simulink model "COMPONENT_model_SEME"  (R2019a)
settings: Solver=ode45  StartTime=0.0  StopTime=60  FixedStep=0.001  RelTol=1e-6  EnableMultiTasking=on
undefined symbols (not defined in the file or in its folder): d, Io, m, pm_0
settings Model: Creator=bhorton  LastModifiedBy=bhorton
settings SolverCC: ZeroCrossAlgorithm=Adaptive
settings DataIOCC: SaveOutput=off  SignalLogging=off  DSMLogging=off  VisualizeSimOutput=off  SaveTime=off  ReturnWorkspaceOutputs=off
settings OptimizationCC: LifeSpan=inf
settings DebuggingCC: AllowSymbolicDim=off  SFUnexpectedBacktrackingDiag=warning  SFNoUnconditionalDefaultTransitionDiag=warning  SFExecutionAtInitializationDiag=none  ArithmeticOperatorsInVariantConditions=warning
settings ModelReferenceCC: PropagateSignalLabelsOutOfModel=off
settings SFSimCC: SimUseLocalCustomCode=off
settings RTWCC: RTWUseLocalCustomCode=off
settings CodeAppCC: StateflowObjectComments=on
settings GRTTargetCC: TargetLangStandard=C89/C90 (ANSI)
settings ConfigComp: CovMetricSettings=dw  CovHtmlReporting=on  CovSaveCumulativeToWorkspaceVar=on  CovSaveSingleToWorkspaceVar=on  CovExternalEMLEnable=off
settings SimscapeCC: SimscapeNormalizeSystem=off

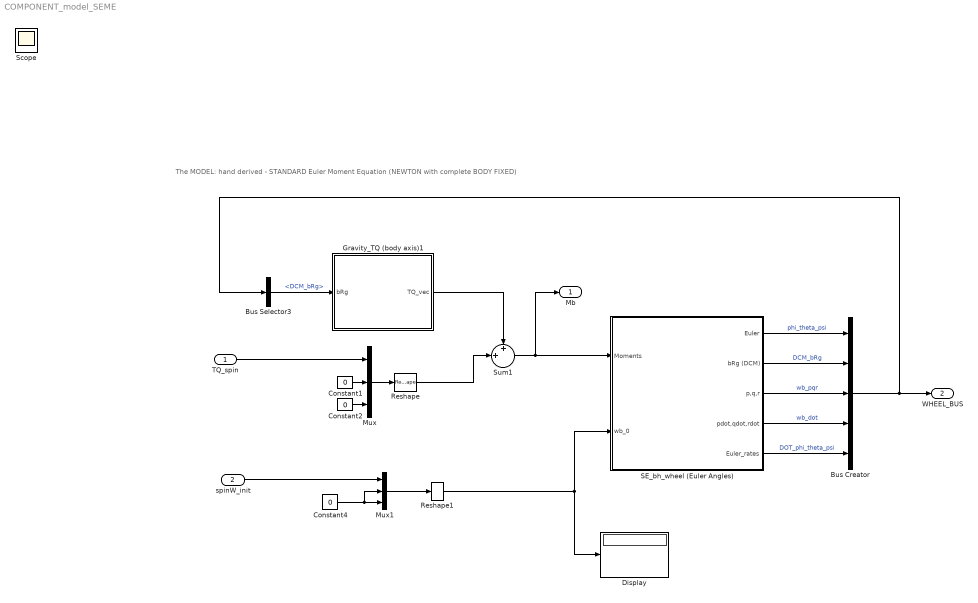
== system COMPONENT_model_SEME ==
  note: The MODEL: hand derived - STANDARD Euler Moment Equation (NEWTON with complete BODY FIXED)
  TQ_spin : Inport
  spinW_init : Inport  Port=2
  Bus Creator : BusCreator  Inputs=5
  Bus Selector3 : BusSelector  OutputSignals=DCM_bRg
  Constant1 : Constant  Value=0
  Constant2 : Constant  Value=0
  Constant4 : Constant  Value=0
  Display : Display
  Gravity_TQ (body axis)1 : Subsystem
  Mux : Mux  Inputs=3
  Mux1 : Mux  Inputs=3
  Reshape : Reshape  OutputDimensionality=Column vector (2-D)
  Reshape1 : Reshape  OutputDimensionality=Column vector (2-D)
  SE_bh_wheel (Euler Angles) : Subsystem  mask(bh_wheel_EoM (Body Axis)){inertia_0=Io, wb_0=[0;0;0], eul_0=deg2rad([0;0;0])}
      mask prompts: inertia_0 "Vehicle Inertia about TOWER pivot point, [kg.m^2]"; wb_0 "Initial body FRAME rotation rates [p,q,r], [rad/sec]"; eul_0 "Initial Euler orientation [yaw, pitch, roll], [rad]"
      mask DialogControl DescTextVar Prompt: Implementation of wheel on a tower equations of motion.
      mask DialogControl Control16 Prompt: Euler angles are used to describe angular pose.
      mask DialogControl Container16 Prompt: PASSIVE rotation sequence
      mask DialogControl Control22 Prompt: The co-ordinate transformation that converts the components of a
      mask DialogControl Control23 Prompt: G-frame vector into its components in the B-frame, is:
      mask DialogControl Control24 Prompt: vb = pR3X(psi) * pR2Y(theta) * pR1Z(phi) * vg
      mask DialogControl Control25 Prompt: vb = bRg * vg
      mask DialogControl Control53 Prompt: You can READ more about PASSIVE rotations, HERE.
      mask DialogControl Control53 Callback: winopen('CONCEPT_PASSIVE_rotations.pdf')
      mask DialogControl Container22 Prompt: ACTIVE rotation sequence
      mask DialogControl Control26 Prompt: To actively reposition (ie: rotate) a B-frame that is initially coincident
      mask DialogControl Control27 Prompt: with the inertial G-frame, into a new pose, we would:
      mask DialogControl Control28 Prompt: vg = inv(pR1Z(phi)) * inv(pR2Y(theta)) * inv(pR3X(psi)) * vb
      mask DialogControl Control30 Prompt: If we define:    aR( ) == inv( pR()  ),  then we can write the above as:
      mask DialogControl Control32 Prompt: vg = aR1Z(phi) * aR2Y(theta) * aR3(psi) * vb
      mask DialogControl Control40 Prompt: You can READ more about ACTIVE rotations, HERE.
      mask DialogControl Control40 Callback: winopen('CONCEPT_ACTIVE_rotations.pdf')
      mask DialogControl Container4 Prompt: Parameters
      mask DialogControl Control11 Prompt: ATTENTION:  note the order of the angles in the list above.
      mask DialogControl Control12 Prompt: This is DIFFERENT to the order used in the Aerospace blockset.
      mask DialogControl Container6 Prompt: DOC
      mask DialogControl Control6 Prompt: In this EULER angle implementation we define the
      mask DialogControl Control7 Prompt: following sequence that rotates a G-frame
      mask DialogControl Control8 Prompt: into a B-frame:
      mask DialogControl Control9_copy Prompt: 1.)  R1Z  : a local rotation about the Z axis by phi, (YAW)
      mask DialogControl Control9_copy_copy Prompt: 2.)  R2Y  : a local rotation about the Y axis by theta, (PITCH)
      mask DialogControl Control17 Prompt: 3.)  R3X  : a local rotation about the X axis by psi, (ROLL)
      mask Display:
      | %port_label('input',1,'{{Mb_{xyz}} (N-m)}','texmode','on');
      | %port_label('output',1,'{\Phi_{Z1} \theta_{Y2} \Psi_{X3} (rad)}','texmode','on');
      | %port_label('output',2,'{DCM bRg }','texmode','on');
      | %port_label('output',3,'{{\omega_b (rad/s)}}','texmode','on');
      | %port_label('output',4,'{{d\omega_b/dt}}','texmode','on');
      | %port_label('output',5,'{d\Phi_{Z1} d\theta_{Y2} d\Psi_{X3} (rad/sec)}','texmode','on');
      | 
      | text(0.5,0.7248,'Body\nEuler Angles','horizontalAlignment','center')
      | text(0.5,0.5048,'WHEEL\nsystem','horizontalAlignment','center')
      | text(0.5,0.3112,'Inertia about\nPIVOT point','horizontalAlignment','center')
  Sum1 : Sum  Inputs=+|+||
  Mb : Outport
  WHEEL_BUS : Outport  Port=2  OutDataTypeStr=Bus: EME_BUS
  Scope : Scope
  wires:
  Constant4/1 -> Mux1/2, Mux1/3
  SE_bh_wheel (Euler Angles)/1(Euler) -> Bus Creator/1  "phi_theta_psi"
  Reshape1/1 -> SE_bh_wheel (Euler Angles)/2(wb_0), Display/1
  Reshape/1 -> Sum1/2
  SE_bh_wheel (Euler Angles)/5(Euler_rates) -> Bus Creator/5  "DOT_phi_theta_psi"
  Bus Creator/1 -> Bus Selector3/1, WHEEL_BUS/1
  spinW_init/1 -> Mux1/1
  Sum1/1 -> SE_bh_wheel (Euler Angles)/1(Moments), Mb/1
  SE_bh_wheel (Euler Angles)/4(pdot,qdot,rdot) -> Bus Creator/4  "wb_dot"
  SE_bh_wheel (Euler Angles)/2(bRg (DCM)) -> Bus Creator/2  "DCM_bRg"
  Gravity_TQ (body axis)1/1(TQ_vec) -> Sum1/1
  Mux1/1 -> Reshape1/1
  SE_bh_wheel (Euler Angles)/3(p,q,r) -> Bus Creator/3  "wb_pqr"
  Bus Selector3/1 -> Gravity_TQ (body axis)1/1(bRg)  "<DCM_bRg>"
  Constant1/1 -> Mux/2
  TQ_spin/1 -> Mux/1
  Constant2/1 -> Mux/3
  Mux/1 -> Reshape/1

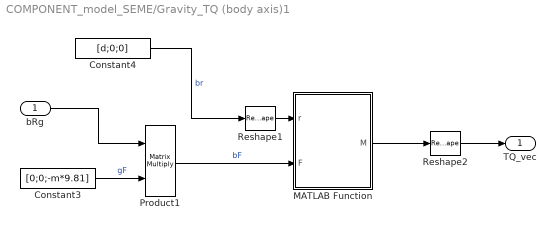
== system COMPONENT_model_SEME/Gravity_TQ (body axis)1 ==
  bRg : Inport
  Constant3 : Constant  Value=[0;0;-m*9.81]  VectorParams1D=off
  Constant4 : Constant  Value=[d;0;0]  VectorParams1D=off
  MATLAB Function : MATLAB Function  TreatAsAtomicUnit=on
  Product1 : Product  Multiplication=Matrix(*)
  Reshape1 : Reshape  OutputDimensionality=Column vector (2-D)
  Reshape2 : Reshape  OutputDimensionality=Column vector (2-D)
  TQ_vec : Outport
  wires:
  Constant3/1 -> Product1/2  "gF"
  bRg/1 -> Product1/1
  Product1/1 -> MATLAB Function/2(F)  "bF"
  Constant4/1 -> Reshape1/1  "br"
  Reshape1/1 -> MATLAB Function/1(r)
  MATLAB Function/1(M) -> Reshape2/1
  Reshape2/1 -> TQ_vec/1

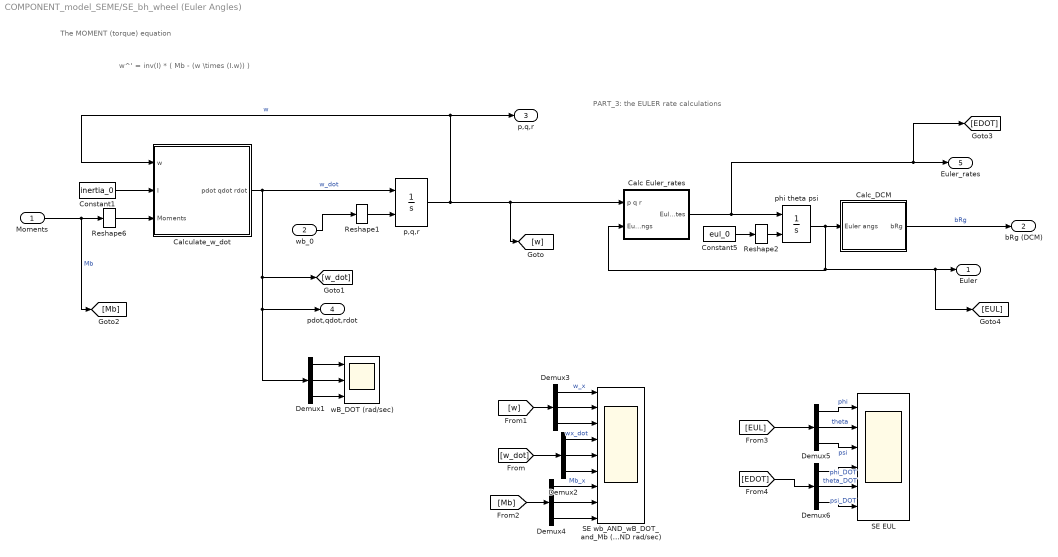
== system COMPONENT_model_SEME/SE_bh_wheel (Euler Angles) ==
  note: w^' = inv(I) * ( Mb - (w \times (I.w)) )
  note: The MOMENT (torque) equation
  note: PART_3: the EULER rate calculations
  Moments : Inport  PortDimensions=3
  wb_0 : Inport  Port=2  PortDimensions=3
  Calc Euler_rates : Subsystem
  Calc_DCM : Subsystem
  Calculate_w_dot : Subsystem
      mask init:
      | %aeroicon('aeroblk');
  Constant1 : Constant  Value=inertia_0  OutDataTypeStr=Inherit: Inherit via back propagation
  Constant5 : Constant  Value=eul_0  OutDataTypeStr=Inherit: Inherit via back propagation
  Demux{1..6} (6 alike) : Demux  Outputs=3
  Reshape1 : Reshape  OutputDimensionality=Column vector (2-D)
  Reshape2 : Reshape  OutputDimensionality=Column vector (2-D)
  Reshape6 : Reshape  OutputDimensionality=Column vector (2-D)
  SE EUL : Scope  NumInputPorts=6
  SE wb_AND_wB_DOT_and_Mb (rad AND rad/sec) : Scope  NumInputPorts=9
  "p,q,r " : Integrator  InitialConditionSource=external  InitialCondition=pm_0
  phi theta psi : Integrator  InitialConditionSource=external  InitialCondition=eul_0
  wB_DOT (rad/sec) : Scope  NumInputPorts=3
  Euler : Outport
  bRg (DCM) : Outport  Port=2
  p,q,r : Outport  Port=3
  pdot,qdot,rdot : Outport  Port=4
  Euler_rates : Outport  Port=5
  wires:
  Moments/1 -> [Mb], Reshape6/1  "Mb"
  Constant1/1 -> Calculate_w_dot/2(I)
  Calculate_w_dot/1(pdot qdot rdot) -> [w_dot], Demux1/1, pdot,qdot,rdot/1, "p,q,r "/1  "w_dot"
  Reshape6/1 -> Calculate_w_dot/3(Moments)
  Reshape1/1 -> "p,q,r "/2
  wb_0/1 -> Reshape1/1
  Demux1/1 -> wB_DOT (rad/sec)/1
  Demux1/2 -> wB_DOT (rad/sec)/2
  Demux1/3 -> wB_DOT (rad/sec)/3
  Reshape2/1 -> phi theta psi/2
  "p,q,r "/1 -> [w], Calc Euler_rates/1("p q r "), Calculate_w_dot/1(w), p,q,r/1  "w"
  Constant5/1 -> Reshape2/1
  Calc Euler_rates/1(Euler_rates) -> phi theta psi/1, [EDOT], Euler_rates/1
  phi theta psi/1 -> Calc Euler_rates/2(Euler_angs), [EUL], Euler/1, Calc_DCM/1(Euler angs)
  Calc_DCM/1(bRg) -> bRg (DCM)/1  "bRg"
  Demux2/2 -> SE wb_AND_wB_DOT_and_Mb (rad AND rad/sec)/5
  Demux3/1 -> SE wb_AND_wB_DOT_and_Mb (rad AND rad/sec)/1  "w_x"
  Demux4/3 -> SE wb_AND_wB_DOT_and_Mb (rad AND rad/sec)/9
  Demux2/3 -> SE wb_AND_wB_DOT_and_Mb (rad AND rad/sec)/6
  Demux3/3 -> SE wb_AND_wB_DOT_and_Mb (rad AND rad/sec)/3
  [Mb] -> Demux4/1
  [w_dot] -> Demux2/1
  [w] -> Demux3/1
  Demux4/1 -> SE wb_AND_wB_DOT_and_Mb (rad AND rad/sec)/7  "Mb_x"
  Demux3/2 -> SE wb_AND_wB_DOT_and_Mb (rad AND rad/sec)/2
  Demux4/2 -> SE wb_AND_wB_DOT_and_Mb (rad AND rad/sec)/8
  Demux2/1 -> SE wb_AND_wB_DOT_and_Mb (rad AND rad/sec)/4  "wx_dot"
  Demux5/2 -> SE EUL/2  "theta"
  Demux5/3 -> SE EUL/3  "psi"
  Demux5/1 -> SE EUL/1  "phi"
  [EUL] -> Demux5/1
  Demux6/2 -> SE EUL/5  "theta_DOT"
  [EDOT] -> Demux6/1
  Demux6/1 -> SE EUL/4  "phi_DOT"
  Demux6/3 -> SE EUL/6  "psi_DOT"

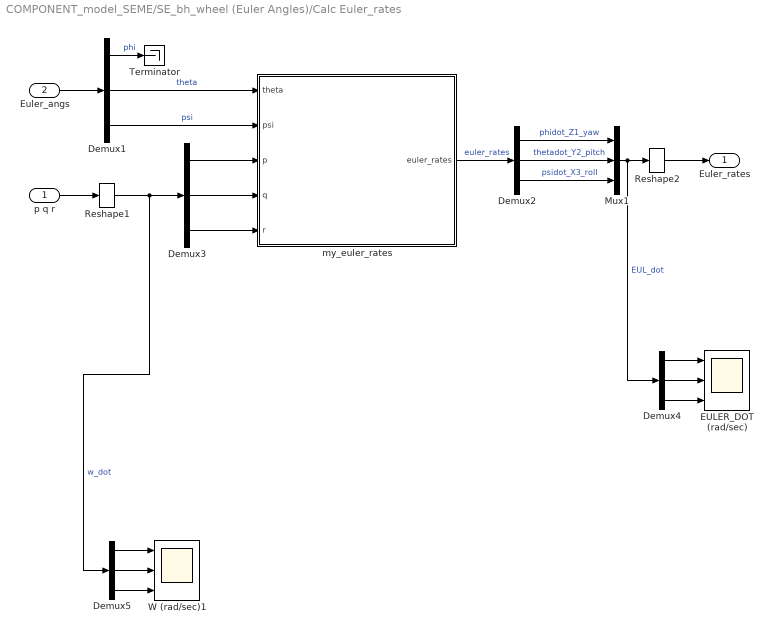
== system COMPONENT_model_SEME/SE_bh_wheel (Euler Angles)/Calc Euler_rates ==
  "p q r " : Inport
  Euler_angs : Inport  Port=2
  Demux{1..5} (5 alike) : Demux  Outputs=3
  EULER_DOT (rad/sec) : Scope  NumInputPorts=3
  Mux1 : Mux  Inputs=3
  Reshape1 : Reshape  OutputDimensionality=Column vector (2-D)
  Reshape2 : Reshape  OutputDimensionality=Column vector (2-D)
  Terminator : Terminator
  W (rad/sec)1 : Scope  NumInputPorts=3
  my_euler_rates : MATLAB Function  TreatAsAtomicUnit=on
  Euler_rates : Outport
  wires:
  my_euler_rates/1(euler_rates) -> Demux2/1  "euler_rates"
  Demux2/3 -> Mux1/3  "psidot_X3_roll"
  Demux2/2 -> Mux1/2  "thetadot_Y2_pitch"
  Demux2/1 -> Mux1/1  "phidot_Z1_yaw"
  Reshape2/1 -> Euler_rates/1
  Demux3/3 -> my_euler_rates/5(r)
  Demux3/2 -> my_euler_rates/4(q)
  Demux3/1 -> my_euler_rates/3(p)
  Euler_angs/1 -> Demux1/1
  "p q r "/1 -> Reshape1/1
  Demux1/2 -> my_euler_rates/1(theta)  "theta"
  Demux1/1 -> Terminator/1  "phi"
  Demux1/3 -> my_euler_rates/2(psi)  "psi"
  Demux4/3 -> EULER_DOT (rad/sec)/3
  Demux4/2 -> EULER_DOT (rad/sec)/2
  Demux4/1 -> EULER_DOT (rad/sec)/1
  Mux1/1 -> Demux4/1, Reshape2/1  "EUL_dot"
  Reshape1/1 -> Demux5/1, Demux3/1  "w_dot"
  Demux5/2 -> W (rad/sec)1/2
  Demux5/1 -> W (rad/sec)1/1
  Demux5/3 -> W (rad/sec)1/3

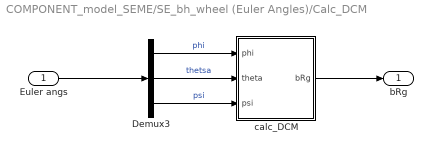
== system COMPONENT_model_SEME/SE_bh_wheel (Euler Angles)/Calc_DCM ==
  Euler angs : Inport
  Demux3 : Demux  Outputs=3
  calc_DCM : MATLAB Function  TreatAsAtomicUnit=on
  bRg : Outport
  wires:
  calc_DCM/1(bRg) -> bRg/1
  Demux3/3 -> calc_DCM/3(psi)  "psi"
  Demux3/2 -> calc_DCM/2(theta)  "thetsa"
  Demux3/1 -> calc_DCM/1(phi)  "phi"
  Euler angs/1 -> Demux3/1

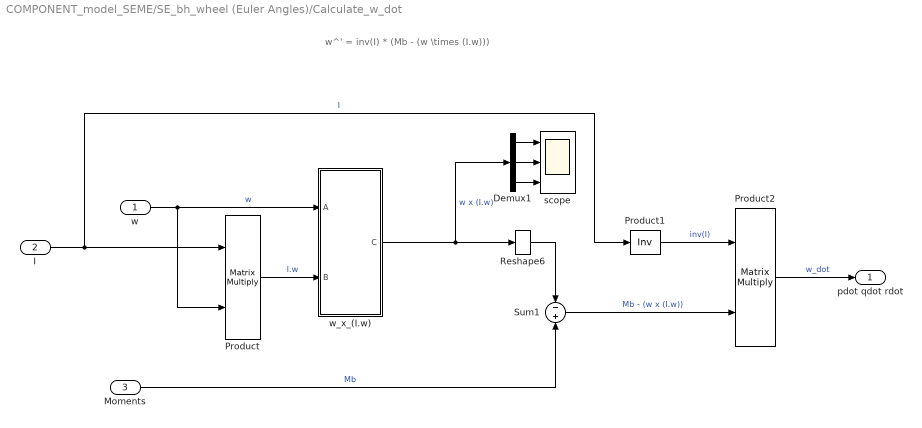
== system COMPONENT_model_SEME/SE_bh_wheel (Euler Angles)/Calculate_w_dot ==
  note: w^' = inv(I) * (Mb - (w \times (I.w)))
  w : Inport
  I : Inport  Port=2
  Moments : Inport  Port=3
  Demux1 : Demux  Outputs=3
  Product : Product  Multiplication=Matrix(*)  SaturateOnIntegerOverflow=on  InputSameDT=on  OutDataTypeStr=Inherit: Same as first input
  Product1 : Product  Inputs=/  Multiplication=Matrix(*)  SaturateOnIntegerOverflow=on  OutDataTypeStr=Inherit: Same as first input
  Product2 : Product  Multiplication=Matrix(*)  SaturateOnIntegerOverflow=on  OutDataTypeStr=Inherit: Same as first input
  Reshape6 : Reshape  OutputDimensionality=Column vector (2-D)
  Sum1 : Sum  Inputs=-|+  SaturateOnIntegerOverflow=on
  scope : Scope  NumInputPorts=3
  w_x_(I.w) : Subsystem
      mask Display:
      | text(.5,.5,'Cross\nProduct\n\nC = AxB', ...
      | 	'HorizontalAlignment','Center',...
      | 	'VerticalAlignment','middle')
  pdot qdot rdot : Outport
  wires:
  w/1 -> w_x_(I.w)/1(A), Product/2  "w"
  Product/1 -> w_x_(I.w)/2(B)  "I.w"
  w_x_(I.w)/1(C) -> Demux1/1, Reshape6/1  "w x (I.w)"
  Product1/1 -> Product2/1  "inv(I)"
  Sum1/1 -> Product2/2  "Mb - (w x (I.w))"
  Product2/1 -> pdot qdot rdot/1  "w_dot"
  Moments/1 -> Sum1/2  "Mb"
  Reshape6/1 -> Sum1/1
  I/1 -> Product/1, Product1/1  "I"
  Demux1/1 -> scope/1
  Demux1/2 -> scope/2
  Demux1/3 -> scope/3

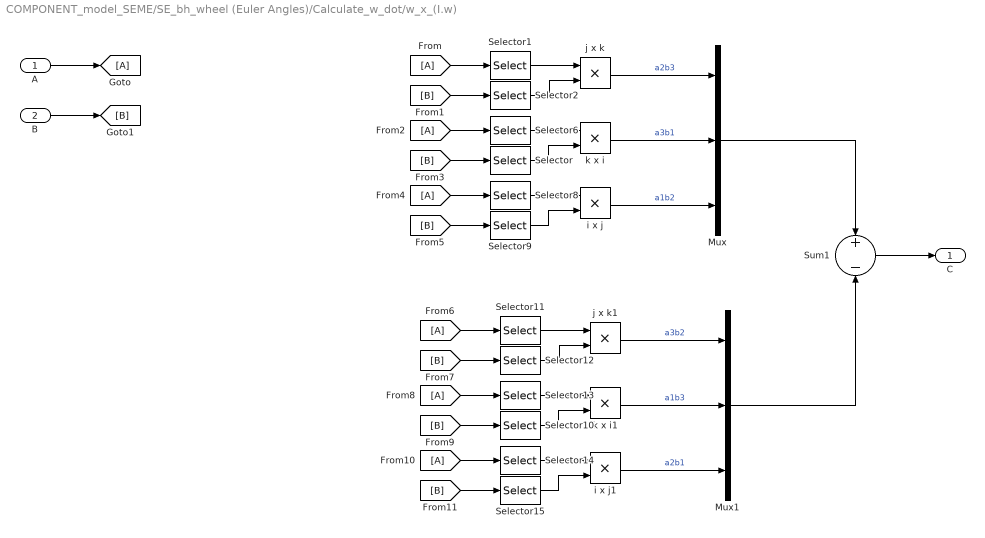
== system COMPONENT_model_SEME/SE_bh_wheel (Euler Angles)/Calculate_w_dot/w_x_(I.w) ==
  A : Inport
  B : Inport  Port=2
  Mux : Mux  Inputs=3
  Mux1 : Mux  Inputs=3
  Selector{,8,13,15} (4 alike) : Selector  InputPortWidth=3  IndexOptions=Index vector (dialog)  Indices=1  OutputSizes=1
  Selector{1,9,12,14} (4 alike) : Selector  InputPortWidth=3  IndexOptions=Index vector (dialog)  Indices=2  OutputSizes=1
  Selector{2,6,10..11} (4 alike) : Selector  InputPortWidth=3  IndexOptions=Index vector (dialog)  Indices=3  OutputSizes=1
  Sum1 : Sum  Inputs=+|-  SaturateOnIntegerOverflow=on  InputSameDT=on  OutDataTypeStr=Inherit: Same as first input
  i x j : Product  SaturateOnIntegerOverflow=on  InputSameDT=on  OutDataTypeStr=Inherit: Same as first input
  i x j1 : Product  SaturateOnIntegerOverflow=on  InputSameDT=on  OutDataTypeStr=Inherit: Same as first input
  j x k : Product  SaturateOnIntegerOverflow=on  InputSameDT=on  OutDataTypeStr=Inherit: Same as first input
  j x k1 : Product  SaturateOnIntegerOverflow=on  InputSameDT=on  OutDataTypeStr=Inherit: Same as first input
  k x i : Product  SaturateOnIntegerOverflow=on  InputSameDT=on  OutDataTypeStr=Inherit: Same as first input
  k x i1 : Product  SaturateOnIntegerOverflow=on  InputSameDT=on  OutDataTypeStr=Inherit: Same as first input
  C : Outport
  wires:
  i x j/1 -> Mux/3  "a1b2"
  k x i/1 -> Mux/2  "a3b1"
  j x k/1 -> Mux/1  "a2b3"
  Mux/1 -> Sum1/1
  Sum1/1 -> C/1
  Selector1/1 -> j x k/1
  Selector2/1 -> j x k/2
  B/1 -> [B]
  A/1 -> [A]
  [B] -> Selector2/1
  [A] -> Selector1/1
  [A] -> Selector6/1
  [B] -> Selector/1
  Selector6/1 -> k x i/1
  Selector/1 -> k x i/2
  [A] -> Selector8/1
  [B] -> Selector9/1
  Selector8/1 -> i x j/1
  Selector9/1 -> i x j/2
  i x j1/1 -> Mux1/3  "a2b1"
  k x i1/1 -> Mux1/2  "a1b3"
  j x k1/1 -> Mux1/1  "a3b2"
  Mux1/1 -> Sum1/2
  Selector11/1 -> j x k1/1
  Selector12/1 -> j x k1/2
  [B] -> Selector12/1
  [A] -> Selector11/1
  [A] -> Selector13/1
  [B] -> Selector10/1
  Selector13/1 -> k x i1/1
  Selector10/1 -> k x i1/2
  [A] -> Selector14/1
  [B] -> Selector15/1
  Selector14/1 -> i x j1/1
  Selector15/1 -> i x j1/2

== matlab function COMPONENT_model_SEME/Gravity_TQ (body axis)1/MATLAB Function ==
  data: r input; M output; F input
function M = cross(r, F)

M = cross(r,F);

== matlab function COMPONENT_model_SEME/SE_bh_wheel (Euler Angles)/Calc Euler_rates/my_euler_rates ==
  data: theta input; euler_rates output; psi input; p input; q input; r input
function euler_rates = my_euler_rates(theta,psi,p,q,r)
%#codegen

%    This function was generated by the Symbolic Math Toolbox version 7.0.
%    09-Jun-2016 10:28:25

euler_rates = [(r.*cos(psi)+q.*sin(psi))./cos(theta);
                q.*cos(psi)-r.*sin(psi);
               (p.*cos(theta)+r.*cos(psi).*sin(theta)+q.*sin(psi).*sin(theta))./cos(theta)];

== matlab function COMPONENT_model_SEME/SE_bh_wheel (Euler Angles)/Calc_DCM/calc_DCM ==
  data: phi input; bRg output; theta input; psi input
function bRg = calc_bRg(phi, theta, psi)
%#codegen

bRg = [ ...
                              cos(phi)*cos(theta),                              cos(theta)*sin(phi),         -sin(theta);
 cos(phi)*sin(psi)*sin(theta) - cos(psi)*sin(phi), cos(phi)*cos(psi) + sin(phi)*sin(psi)*sin(theta), cos(theta)*sin(psi);
 sin(phi)*sin(psi) + cos(phi)*cos(psi)*sin(theta), cos(psi)*sin(phi)*sin(theta) - cos(phi)*sin(psi), cos(psi)*cos(theta);
 ];

end
